simulink model "Lithium_ion_cell_1RC_1800mAh"  (R2020a)
settings: Solver=VariableStepAuto  StartTime=0.0  StopTime=42500  RelTol=1e-3
undefined symbols (not defined in the file): C1, C_nom, I_table, OCV, R1, Rs, SOC_parameters
libraries: nesl_utility x8, fl_lib x7, ee_lib x1
settings Model: OrderedModelArguments=off  Creator=thibaultnouvellon  LastModifiedBy=thibaultnouvellon

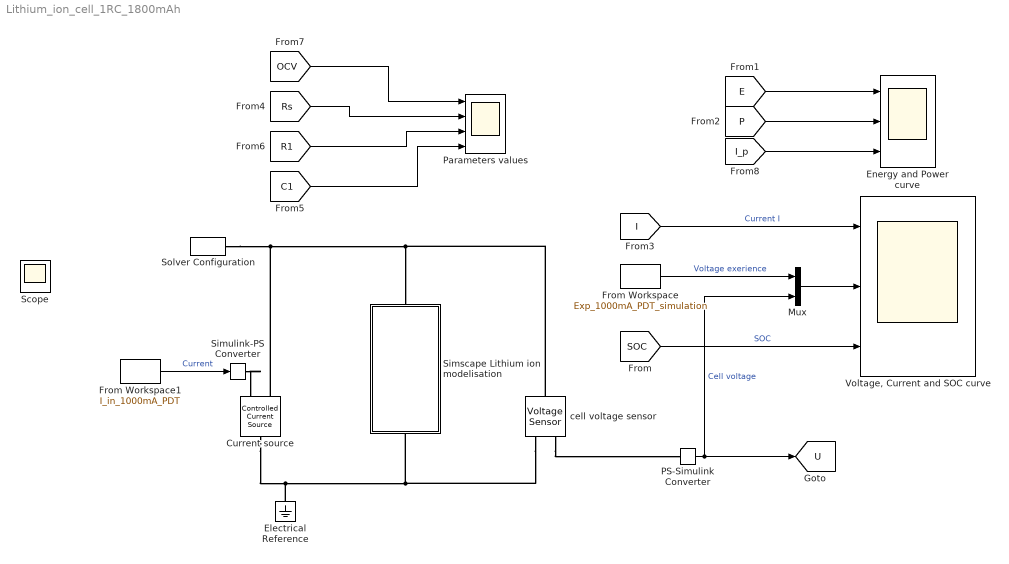
== system Lithium_ion_cell_1RC_1800mAh ==
  Current source : fl_lib/Electrical/Electrical Sources/Controlled Current Source
  Electrical Reference : fl_lib/Electrical/Electrical Elements/Electrical Reference
  Energy and Power curve : Scope  NumInputPorts=3
  From Workspace : FromWorkspace  VariableName=Exp_1000mA_PDT_simulation  SampleTime=1
  From Workspace1 : FromWorkspace  VariableName=I_in_1000mA_PDT  SampleTime=1
  Mux : Mux  Inputs=2
  PS-Simulink Converter : nesl_utility/PS-Simulink Converter  PhysicalDomain=network_engine_domain  SubClassName=ps_output  LeftPortType=input  RightPortType=output  PseudoPeriodic=off  Frequencies=[]  Unit=inherit  AffineConversion=off
  Parameters values : Scope  NumInputPorts=4
  Simscape Lithium ion modelisation : Subsystem
  Simulink-PS Converter : nesl_utility/Simulink-PS Converter  PhysicalDomain=network_engine_domain  SubClassName=ps_input  LeftPortType=input  RightPortType=output  PseudoPeriodic=off  Frequencies=[]  NoiseDistribution=none  NoiseParameters=[]  Unit=1  AffineConversion=off  FilteringAndDerivatives=provide  SimscapeFilterOrder=1  InputFilterTimeConstant=0.001  UdotUserProvided=0
  Solver Configuration : nesl_utility/Solver Configuration  PhysicalDomain=network_engine_domain  SubClassName=solver  LeftPortType=input  RightPortType=generic  Tones=[]  Harmonics=[]  SimulateNoise=off  Profile=off  UseLocalSampling=off  EnableSwitchedLinearOptims=on  FrequencyDomain=off  UseCCode=off  RelTol=0.001  AbsTol=1e-06  MinStep=1e-09  ToWorkspace=off  RevertToSquareIcSolve=off  NumHomotopyIterations=100  PhasorMode=off  PhasorModeNumHarmonics=1  DoDC=off  ResidualTolerance=1e-09  UseLocalSolver=off  LocalSolverChoice=NE_BACKWARD_EULER_ADVANCER  LocalSolverSampleTime=0.001  DoFixedCost=off  MaxNonlinIter=3  MaxModeIter=2  LinearAlgebra=auto  EquationFormulation=NE_TIME_EF  DelaysMemoryBudget=1024  AutomaticFiltering=on  FilteringTimeConstant=0.001  PartitionStorageMethod=AS_NEEDED  PartitionMemoryBudget=1024  PartitionMethod=ROBUST
  "Voltage, Current and SOC curve" : Scope  NumInputPorts=3
  cell voltage sensor : fl_lib/Electrical/Electrical Sensors/Voltage Sensor
  Scope : Scope
  tag scope: U=global
  wires:
  PS-Simulink Converter/1 -> [U], Mux/2  "Cell voltage"
  From Workspace/1 -> Mux/1  "Voltage exerience"
  [SOC] -> "Voltage, Current and SOC curve"/3  "SOC"
  Mux/1 -> "Voltage, Current and SOC curve"/2
  From Workspace1/1 -> Simulink-PS Converter/1  "Current"
  [R1] -> Parameters values/3
  [C1] -> Parameters values/4
  [OCV] -> Parameters values/1
  [Rs] -> Parameters values/2
  [I] -> "Voltage, Current and SOC curve"/1  "Current I"
  [P] -> Energy and Power curve/2
  [I_p] -> Energy and Power curve/3
  [E] -> Energy and Power curve/1
  connections:
  Electrical Reference/LConn1 -- Current source/LConn1 -- cell voltage sensor/RConn2 -- Simscape Lithium ion modelisation/RConn1
  Solver Configuration/RConn1 -- cell voltage sensor/LConn1 -- Simscape Lithium ion modelisation/LConn1 -- Current source/RConn2
  cell voltage sensor/RConn1 -- PS-Simulink Converter/LConn1
  Simulink-PS Converter/RConn1 -- Current source/RConn1

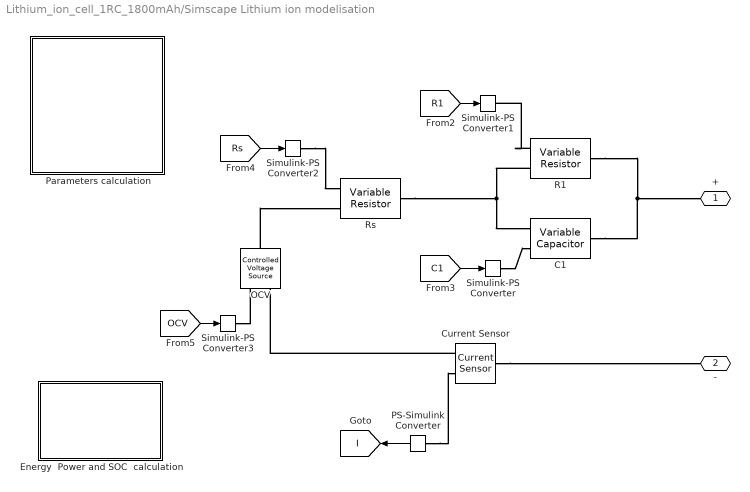
== system Lithium_ion_cell_1RC_1800mAh/Simscape Lithium ion modelisation ==
  " OCV" : fl_lib/Electrical/Electrical Sources/Controlled Voltage Source
  C1 : ee_lib/Passive/Variable Capacitor  prm=2  Cmin=1e-9 F  r=1e-6 Ohm  v0=0 V  q0=0 C
      settings: SourceProductBaseCode=PS  InternalSimscapePortConfiguration="{\"Bottom\":[],\"Left\":[{\"id\":\"C\",\"label\":\"C\",\"type\":\"input\"},{\"id\":\"p\",\"label\":\"+\",\"type\":\"foundation.electrical.electrical\"}],\"Right\":[{\"id\":\"n\",\"label\":\"-\",\"type\":\"foundation.electrical.electrical\"}],\"Top\":[]}"
  Current Sensor : fl_lib/Electrical/Electrical Sensors/Current Sensor
  Energy  Power and SOC  calculation : Subsystem
  PS-Simulink Converter : nesl_utility/PS-Simulink Converter  PhysicalDomain=network_engine_domain  SubClassName=ps_output  LeftPortType=input  RightPortType=output  PseudoPeriodic=off  Frequencies=[]  Unit=inherit  AffineConversion=off
  Parameters calculation : Subsystem
  R1 : fl_lib/Electrical/Electrical Elements/Variable Resistor  Rmin=0 Ohm  i_specify=off  i_priority=None  i=0 A  i_nominal_specify=off  i_nominal_unit=A  i_nominal_value=1  v_specify=off  v_priority=None  v=0 V  v_nominal_specify=off  v_nominal_unit=V  v_nominal_value=1
  Rs : fl_lib/Electrical/Electrical Elements/Variable Resistor  Rmin=0 Ohm  i_specify=off  i_priority=None  i=0 A  i_nominal_specify=off  i_nominal_unit=A  i_nominal_value=1  v_specify=off  v_priority=None  v=0 V  v_nominal_specify=off  v_nominal_unit=V  v_nominal_value=1
  Simulink-PS Converter{,1..3} (4 alike) : nesl_utility/Simulink-PS Converter  PhysicalDomain=network_engine_domain  SubClassName=ps_input  LeftPortType=input  RightPortType=output  PseudoPeriodic=off  Frequencies=[]  NoiseDistribution=none  NoiseParameters=[]  Unit=1  AffineConversion=off  FilteringAndDerivatives=provide  SimscapeFilterOrder=1  InputFilterTimeConstant=0.001  UdotUserProvided=0
  + : PMIOPort  Side=Left
  - : PMIOPort  Port=2  Side=Right
  tag scope: I=global
  wires:
  PS-Simulink Converter/1 -> [I]
  [R1] -> Simulink-PS Converter1/1
  [Rs] -> Simulink-PS Converter2/1
  [C1] -> Simulink-PS Converter/1
  [OCV] -> Simulink-PS Converter3/1
  connections:
  R1/LConn2 -- Rs/RConn1 -- C1/LConn2
  Simulink-PS Converter/RConn1 -- C1/LConn1
  " OCV"/LConn1 -- Rs/LConn2
  Simulink-PS Converter2/RConn1 -- Rs/LConn1
  Simulink-PS Converter3/RConn1 -- " OCV"/RConn1
  R1/LConn1 -- Simulink-PS Converter1/RConn1
  C1/RConn1 -- R1/RConn1 -- +/RConn1
  Current Sensor/LConn1 -- -/RConn1
  Current Sensor/RConn2 -- " OCV"/RConn2
  PS-Simulink Converter/LConn1 -- Current Sensor/RConn1

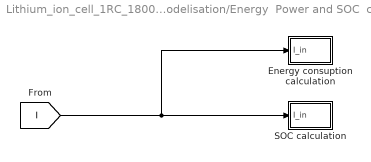
== system Lithium_ion_cell_1RC_1800mAh/Simscape Lithium ion modelisation/Energy  Power and SOC  calculation ==
  Energy consuption calculation : Subsystem
  SOC calculation : Subsystem
  wires:
  [I] -> Energy consuption calculation/1(I_in), SOC calculation/1(I_in)

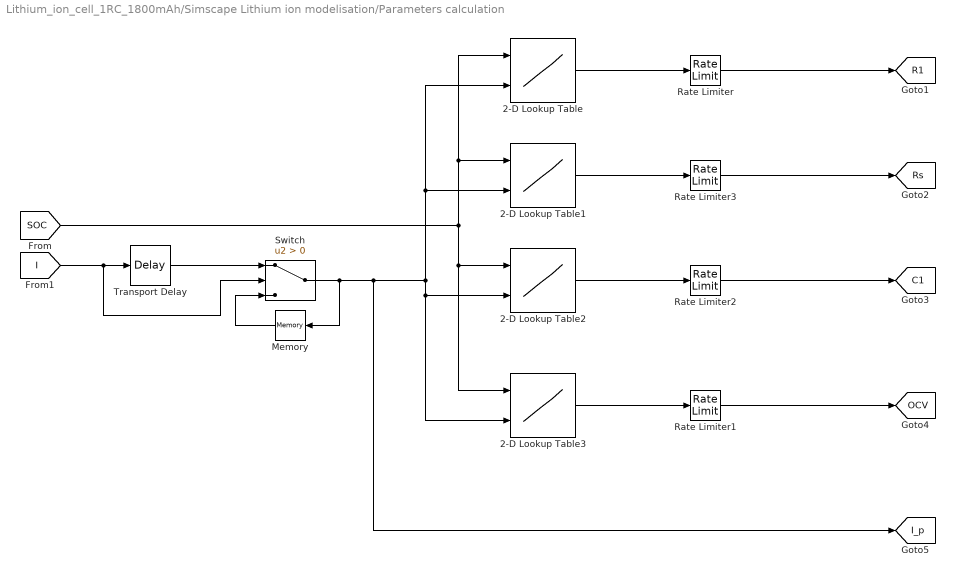
== system Lithium_ion_cell_1RC_1800mAh/Simscape Lithium ion modelisation/Parameters calculation ==
  2-D Lookup Table : Lookup_n-D  BreakpointsForDimension1=SOC_parameters  BreakpointsForDimension2=I_table  Table=R1  InternalRulePriority=Speed  RndMeth=Simplest  InputSameDT=on
  2-D Lookup Table1 : Lookup_n-D  BreakpointsForDimension1=SOC_parameters  BreakpointsForDimension2=I_table  Table=Rs  InternalRulePriority=Speed  RndMeth=Simplest  InputSameDT=on
  2-D Lookup Table2 : Lookup_n-D  BreakpointsForDimension1=SOC_parameters  BreakpointsForDimension2=I_table  Table=C1  InternalRulePriority=Speed  RndMeth=Simplest  InputSameDT=on
  2-D Lookup Table3 : Lookup_n-D  BreakpointsForDimension1=SOC_parameters  BreakpointsForDimension2=I_table  Table=OCV  InternalRulePriority=Speed  RndMeth=Simplest  InputSameDT=on
  Memory : Memory
  Rate Limiter : RateLimiter  RisingSlewLimit=10^(-3)  FallingSlewLimit=-10^(-3)  SampleTimeMode=inherited
  Rate Limiter1 : RateLimiter  RisingSlewLimit=10^(-3)  FallingSlewLimit=-10^(-3)  SampleTimeMode=inherited
  Rate Limiter2 : RateLimiter  RisingSlewLimit=10^(-2)  FallingSlewLimit=-10^(-2)  SampleTimeMode=inherited
  Rate Limiter3 : RateLimiter  RisingSlewLimit=10^(-3)  FallingSlewLimit=-10^(-3)  SampleTimeMode=inherited
  Switch : Switch  Criteria=u2 > Threshold
  Transport Delay : TransportDelay  DelayTime=2
  tag scope: C1=global, I_p=global, OCV=global, R1=global, Rs=global
  wires:
  [SOC] -> 2-D Lookup Table1/1, 2-D Lookup Table/1, 2-D Lookup Table2/1, 2-D Lookup Table3/1
  2-D Lookup Table1/1 -> Rate Limiter3/1
  2-D Lookup Table3/1 -> Rate Limiter1/1
  Memory/1 -> Switch/3
  Transport Delay/1 -> Switch/1
  2-D Lookup Table2/1 -> Rate Limiter2/1
  Switch/1 -> Memory/1, [I_p], 2-D Lookup Table/2, 2-D Lookup Table1/2, 2-D Lookup Table3/2, 2-D Lookup Table2/2
  [I] -> Transport Delay/1, Switch/2
  2-D Lookup Table/1 -> Rate Limiter/1
  Rate Limiter/1 -> [R1]
  Rate Limiter3/1 -> [Rs]
  Rate Limiter2/1 -> [C1]
  Rate Limiter1/1 -> [OCV]

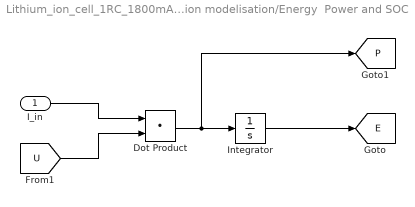
== system Lithium_ion_cell_1RC_1800mAh/Simscape Lithium ion modelisation/Energy  Power and SOC  calculation/Energy consuption calculation ==
  I_in : Inport
  Dot Product : DotProduct  InputSameDT=on  OutDataTypeStr=Inherit: Inherit via internal rule
  Integrator : Integrator
  tag scope: E=global, P=global
  wires:
  Integrator/1 -> [E]
  [U] -> Dot Product/2
  I_in/1 -> Dot Product/1
  Dot Product/1 -> [P], Integrator/1

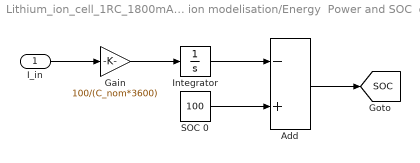
== system Lithium_ion_cell_1RC_1800mAh/Simscape Lithium ion modelisation/Energy  Power and SOC  calculation/SOC calculation ==
  I_in : Inport
  Add : Sum  Inputs=-+
  Gain : Gain  Gain=100/(C_nom*3600)
  Integrator : Integrator
  SOC 0 : Constant  Value=100
  tag scope: SOC=global
  wires:
  I_in/1 -> Gain/1
  Gain/1 -> Integrator/1
  Integrator/1 -> Add/1
  Add/1 -> [SOC]
  SOC 0/1 -> Add/2
